simulink model "lab4_symulacja"  (R2022a)
settings: Solver=VariableStepAuto  StartTime=0.0  StopTime=50.0  RelTol=1e-3
values from neighbouring files (symbols this model uses):
  ki = 1    [lab4.m]
  kp = 7    [lab4.m]
settings Model: Creator=rober  LastModifiedBy=rober

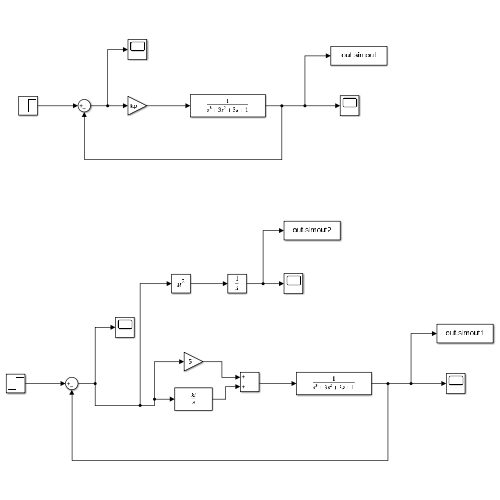
[thumbnail: Simulink's stored preview of the top-level diagram]
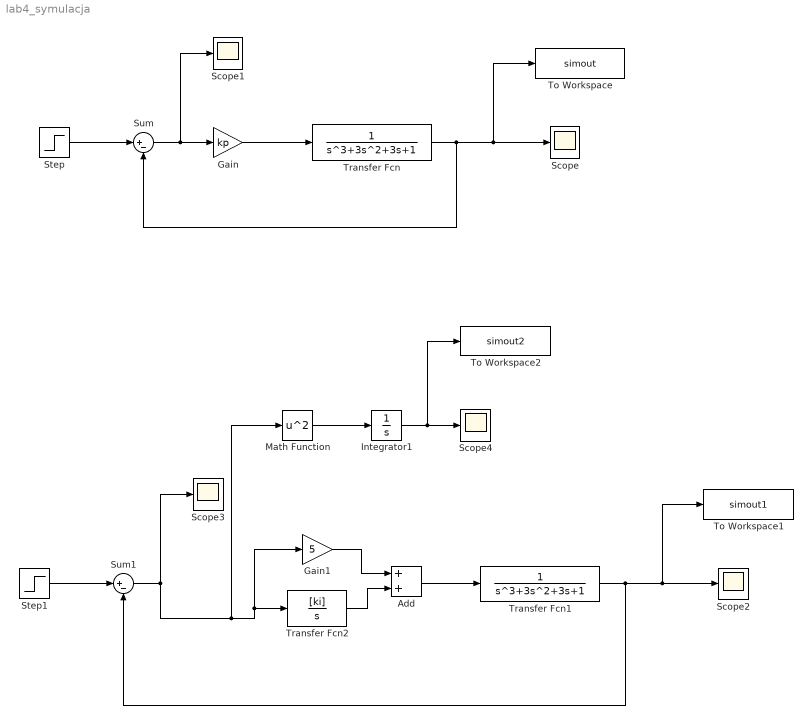
== system lab4_symulacja ==
  Add : Sum
  Gain : Gain  Gain=kp
  Gain1 : Gain  Gain=5
  Integrator1 : Integrator
  Math Function : Math  Operator=square
  Scope{,1..4} (5 alike) : Scope
  Step : Step  SampleTime=0
  Step1 : Step  SampleTime=0
  Sum : Sum  Inputs=|+-
  Sum1 : Sum  Inputs=|+-
  To Workspace : ToWorkspace  VariableName=simout  SampleTime=-1
  To Workspace1 : ToWorkspace  VariableName=simout1  SampleTime=-1
  To Workspace2 : ToWorkspace  VariableName=simout2  SampleTime=-1
  Transfer Fcn : TransferFcn  Denominator=[1 3 3 1]
  Transfer Fcn1 : TransferFcn  Denominator=[1 3 3 1]
  Transfer Fcn2 : TransferFcn  Numerator=[ki]  Denominator=[1 0]
  wires:
  Gain/1 -> Transfer Fcn/1
  Step/1 -> Sum/1
  Sum/1 -> Scope1/1, Gain/1
  Transfer Fcn/1 -> Sum/2, To Workspace/1, Scope/1
  Step1/1 -> Sum1/1
  Transfer Fcn1/1 -> Sum1/2, To Workspace1/1, Scope2/1
  Sum1/1 -> Math Function/1, Transfer Fcn2/1, Gain1/1, Scope3/1
  Add/1 -> Transfer Fcn1/1
  Gain1/1 -> Add/1
  Transfer Fcn2/1 -> Add/2
  Math Function/1 -> Integrator1/1
  Integrator1/1 -> To Workspace2/1, Scope4/1
